simulink model "simulation_control_observerLQR_NL_WP3"  (R2023b)
settings: Solver=VariableStepAuto  StartTime=0.0  StopTime=20  RelTol=1e-3
values from neighbouring files (symbols this model uses):
  A = [0 1; 9.81 -0.1]    [WP3.m]
  B = [0; 1]    [WP3.m]
  C = [1 0]    [WP3.m]
  K = [92.0469   14.4179]    [WP3.m]
  L = [l1; l2]    [WP3.m]
settings Model: Creator=giova  LastModifiedBy=giova

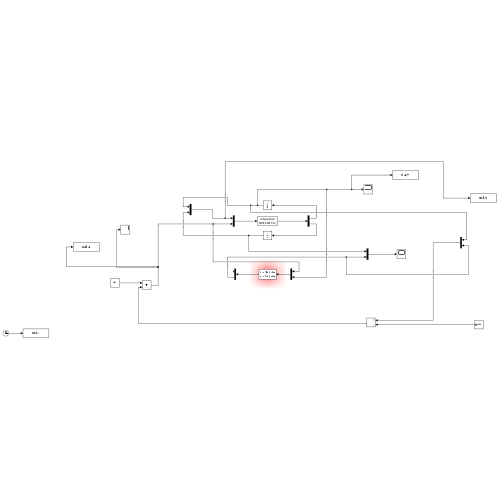
[thumbnail: Simulink's stored preview of the top-level diagram]
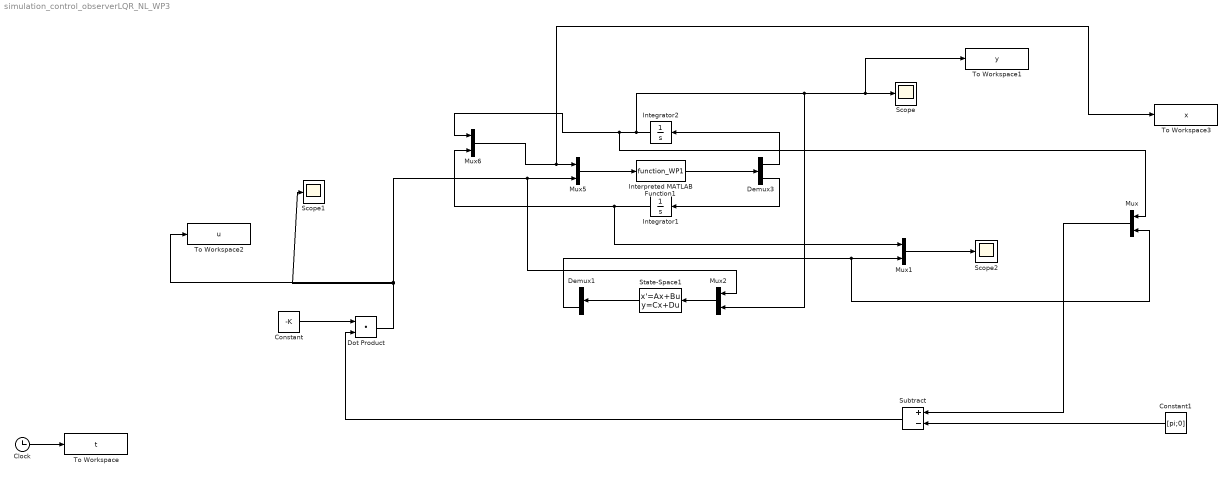
== system simulation_control_observerLQR_NL_WP3 ==
  Clock : Clock
  Constant : Constant  Value=-K
  Constant1 : Constant  Value=[pi;0]
  Demux1 : Demux  Outputs=2
  Demux3 : Demux  Outputs=2
  Dot Product : DotProduct  OutDataTypeStr=Inherit: Inherit via internal rule
  Integrator1 : Integrator
  Integrator2 : Integrator
  Interpreted MATLAB Function1 : MATLABFcn  MATLABFcn=function_WP1  OutputDimensions=2
  Mux{,1..2,5..6} (5 alike) : Mux  Inputs=2
  Scope : Scope
  Scope1 : Scope
  Scope2 : Scope
  State-Space1 : StateSpace  A=A-L*C  B=[B L]  C=eye(2)  D=[0 0; 0 0]  InitialCondition=[0 0]
  Subtract : Sum  Inputs=+-
  To Workspace : ToWorkspace  VariableName=t  SampleTime=-1
  To Workspace1 : ToWorkspace  VariableName=y  SampleTime=-1
  To Workspace2 : ToWorkspace  VariableName=u  SampleTime=-1
  To Workspace3 : ToWorkspace  VariableName=x  SampleTime=-1
  wires:
  State-Space1/1 -> Demux1/1
  Clock/1 -> To Workspace/1
  Integrator1/1 -> Mux1/1, Mux6/2
  Mux5/1 -> Interpreted MATLAB Function1/1
  Interpreted MATLAB Function1/1 -> Demux3/1
  Mux2/1 -> State-Space1/1
  Mux6/1 -> To Workspace3/1, Mux5/1
  Demux3/2 -> Integrator1/1
  Demux3/1 -> Integrator2/1
  Integrator2/1 -> Mux2/2, To Workspace1/1, Scope/1, Mux6/1, Mux/1
  Demux1/2 -> Mux/2, Mux1/2
  Mux1/1 -> Scope2/1
  Constant1/1 -> Subtract/2
  Constant/1 -> Dot Product/1
  Subtract/1 -> Dot Product/2
  Dot Product/1 -> To Workspace2/1, Mux2/1, Mux5/2, Scope1/1
  Mux/1 -> Subtract/1
